simulink model "fByFullMatlab"  (R2016b)
settings: Solver=FixedStepDiscrete  StartTime=0.0  StopTime=10.0  RelTol=1e-3
settings Model: DataTypeOverride=Off  Creator=hasee  LastModifiedBy=hasee
settings DataIOCC: LimitDataPoints=on  SaveOutput=off  SaveTime=off
settings OptimizationCC: BlockReduction=off  ConditionallyExecuteInputs=off  DefaultParameterBehavior=Inlined  LifeSpan=inf
settings DebuggingCC: AlgebraicLoopMsg=error  SingleTaskRateTransMsg=error  AllowSymbolicDim=off  StrictBusMsg=ErrorOnBusTreatedAsVector  SFUnexpectedBacktrackingDiag=warning  SFNoUnconditionalDefaultTransitionDiag=warning  SFExecutionAtInitializationDiag=none
settings HardwareCC: ProdBitPerPointer=32  ProdBitPerSizeT=32  ProdBitPerPtrDiffT=32  ProdLargestAtomicFloat=None  ProdIntDivRoundTo=Undefined  ProdEndianess=Unspecified  ProdWordSize=32  ProdHWDeviceType=ASIC/FPGA->ASIC/FPGA  ProdEqTarget=off
settings GRTTargetCC: TargetLangStandard=C89/C90 (ANSI)  GeneratePreprocessorConditionals=Disable all
settings ConfigComp: CovScope=ReferencedModels  CovMetricSettings=dw  CovHtmlReporting=on  CovSaveCumulativeToWorkspaceVar=on  CovSaveSingleToWorkspaceVar=on  CovExternalEMLEnable=off  CovSFcnEnable=off

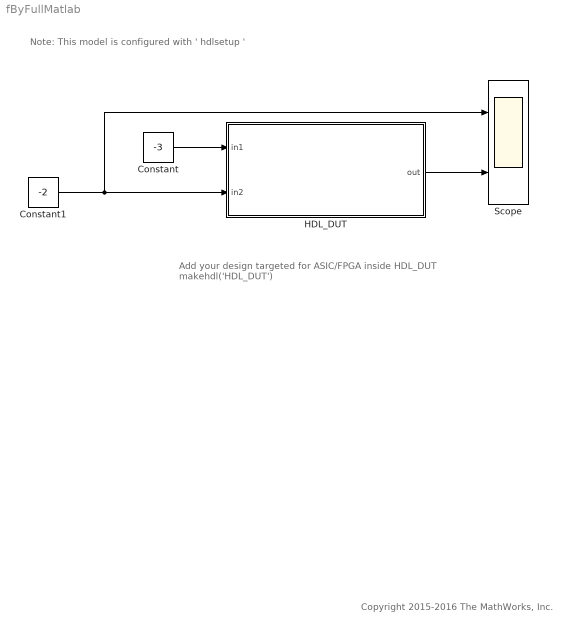
== system fByFullMatlab ==
  note: Note: This model is configured with ' hdlsetup '
  note: Add your design targeted for ASIC/FPGA inside HDL_DUT
      | makehdl('HDL_DUT')
  note: Copyright 2015-2016 The MathWorks, Inc.
  Constant : Constant  Value=-3  OutDataTypeStr=int8  SampleTime=-1
  Constant1 : Constant  Value=-2  OutDataTypeStr=int8  SampleTime=-1
  HDL_DUT : Subsystem
  Scope : Scope  NumInputPorts=2
  wires:
  Constant/1 -> HDL_DUT/1(in1)
  Constant1/1 -> Scope/1, HDL_DUT/2(in2)
  HDL_DUT/1(out) -> Scope/2

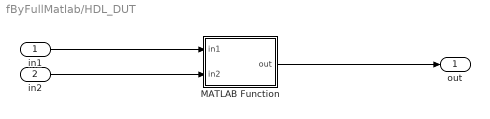
== system fByFullMatlab/HDL_DUT ==
  in1 : Inport
  in2 : Inport  Port=2
  MATLAB Function : MATLAB Function  TreatAsAtomicUnit=on
  out : Outport
  wires:
  in1/1 -> MATLAB Function/1(in1)
  in2/1 -> MATLAB Function/2(in2)
  MATLAB Function/1(out) -> out/1

== matlab function fByFullMatlab/HDL_DUT/MATLAB Function ==
  data: in1 input; out output; in2 input
function out = fcn(in1, in2)
%#codegen
if (in1>0 && in2>0) ||(in1<0 && in2<0)
    out=min(abs(in1),abs(in2));
else
    out=-min(abs(in1),abs(in2));
end
